simulink model "compute_topo_ini"  (R2014b)
settings: Solver=ode3  StartTime=0.0  StopTime=120  FixedStep=0.04  RelTol=1e-3
undefined symbols (not defined in the file or in its folder): cfe_initial_utc_time, ini_position_v, ini_velocity_v
libraries: telem_conversion_lib x1
settings Model: Creator=Jim Kaidy  LastModifiedBy=mstewart
settings DataIOCC: SignalLoggingSaveFormat=ModelDataLogs
settings OptimizationCC: ExpressionDepthLimit=2147483647
settings DebuggingCC: UnderspecifiedInitializationDetection=Classic  MergeDetectMultiDrivingBlocksExec=none  FcnCallInpInsideContextMsg=EnableAllAsWarning  StateNameClashWarn=warning

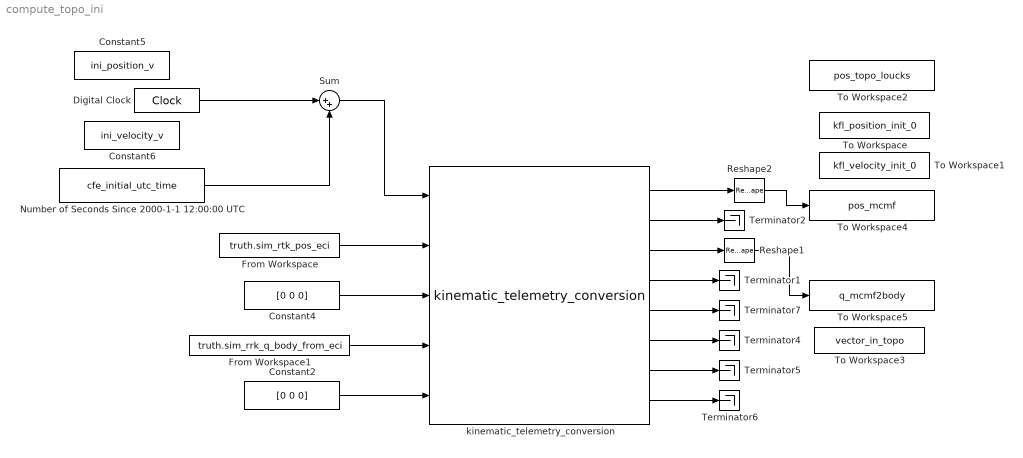
== system compute_topo_ini ==
  Constant2 : Constant  Value=[0 0 0]
  Constant4 : Constant  Value=[0 0 0]
  Constant5 : Constant  Value=ini_position_v
  Constant6 : Constant  Value=ini_velocity_v
  Digital Clock : DigitalClock  SampleTime=0.04
  From Workspace : FromWorkspace  VariableName=truth.sim_rtk_pos_eci  SampleTime=0
  From Workspace1 : FromWorkspace  VariableName=truth.sim_rrk_q_body_from_eci  SampleTime=0
  Number of Seconds Since 2000-1-1 12:00:00 UTC : Constant  Description=|  Value=cfe_initial_utc_time
      | Number of Seconds                   
      | July 4, 2014 22:40:00 UTC           
      | Calculate on Web Site:              
      | www.mbari.org/staff/rich/utccalc.htm
  Reshape1 : Reshape
  Reshape2 : Reshape
  Sum : Sum  Inputs=|++
  Terminator{1..2,4..7} (6 alike) : Terminator
  To Workspace : ToWorkspace  VariableName=kfl_position_init_0  SampleTime=-1
      settings: MaxDataPoints=1
  To Workspace1 : ToWorkspace  VariableName=kfl_velocity_init_0  SampleTime=-1
      settings: MaxDataPoints=1
  To Workspace2 : ToWorkspace  VariableName=pos_topo_loucks  SaveFormat=Timeseries  SampleTime=-1
  To Workspace3 : ToWorkspace  VariableName=vector_in_topo  SampleTime=-1
      settings: MaxDataPoints=1
  To Workspace4 : ToWorkspace  VariableName=pos_mcmf  SaveFormat=Timeseries  SampleTime=-1
  To Workspace5 : ToWorkspace  VariableName=q_mcmf2body  SaveFormat=Timeseries  SampleTime=-1
  kinematic_telemetry_conversion : telem_conversion_lib/kinematic_telemetry_conversion
  wires:
  From Workspace1/1 -> kinematic_telemetry_conversion/4
  kinematic_telemetry_conversion/1 -> Reshape2/1
  kinematic_telemetry_conversion/2 -> Terminator2/1
  kinematic_telemetry_conversion/3 -> Reshape1/1
  kinematic_telemetry_conversion/6 -> Terminator4/1
  kinematic_telemetry_conversion/7 -> Terminator5/1
  Constant2/1 -> kinematic_telemetry_conversion/5
  kinematic_telemetry_conversion/8 -> Terminator6/1
  kinematic_telemetry_conversion/5 -> Terminator7/1
  kinematic_telemetry_conversion/4 -> Terminator1/1
  Number of Seconds Since 2000-1-1 12:00:00 UTC/1 -> Sum/2
  Digital Clock/1 -> Sum/1
  Sum/1 -> kinematic_telemetry_conversion/1
  Reshape1/1 -> To Workspace5/1
  Reshape2/1 -> To Workspace4/1
  From Workspace/1 -> kinematic_telemetry_conversion/2
  Constant4/1 -> kinematic_telemetry_conversion/3
